simulink library "firstOrderDiscreteTimeFilter"  (R2018a)
settings: Solver=VariableStepAuto  StartTime=0.0  StopTime=10.0  RelTol=1e-3
undefined symbols (not defined in the file): ctrl, DiscIntNeverNeededParam
settings Model: Creator=M.Cobb  LastModifiedBy=M.Cobb

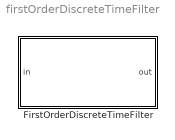
== system firstOrderDiscreteTimeFilter ==
  FirstOrderDiscreteTimeFilter : Subsystem

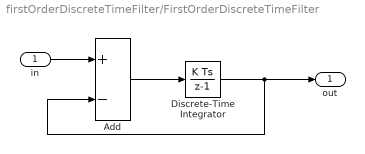
== system firstOrderDiscreteTimeFilter/FirstOrderDiscreteTimeFilter ==
  in : Inport
  Add : Sum  Inputs=+-
  Discrete-Time Integrator : DiscreteIntegrator  gainval=1/ctrl.reelSpeedTimeConstant  InitialCondition=ctrl.initialReelSpeed  SampleTime=-1  ICPrevOutput=DiscIntNeverNeededParam  ICPrevScaledInput=DiscIntNeverNeededParam
  out : Outport
  wires:
  in/1 -> Add/1
  Add/1 -> Discrete-Time Integrator/1
  Discrete-Time Integrator/1 -> Add/2, out/1
